simulink model "sim_Aircraft_f"  (R2016b)
settings: Solver=VariableStepAuto  StartTime=0.0  StopTime=230.0  RelTol=1e-3
values from neighbouring files (symbols this model uses):
  A = [-0.322, 0.052, 0.028, -1.12 , 0.002;       0     , 0    , 1    , -0.001,     0;       -10.6 , 0    , -2.87, 0.46  , -0.65;       6.87  , 0    , -0.04, -0.32 , -0.02;       0     , 0    , 0    , 0     ,   -10 ]    [run_task_3f.m]
  A_k = [-0.322, 0.052, 0.028, -1.12 ;       0     , 0    , 1    , -0.001;       -10.6 , 0    , -2.87, 0.46  ;       6.87  , 0    , -0.04, -0.32]    [run_task_3f.m]
  B = [0 0 0 0 10]'    [run_task_3f.m]
  B_k = [0.002, 0, -0.65, -0.2]'    [run_task_3f.m]
  C = [0 0 0 1 0;       0 0 1 0 0;       1 0 0 0 0;       0 1 0 0 0]    [run_task_3f.m]
  C_k = [0 1 0 0;       0 0 1 0;       0 0 0 1]    [run_task_3f.m]
  D = zeros(4,1)    [run_task_3f.m]
  D_k = zeros(3,1)    [run_task_3f.m]
  k_d_phi = f_kd(zp, wp)    [run_task_3f.m]
  k_i_chi = V_g/g * wx^2    [run_task_3f.m]
  k_i_phi = 0    [run_task_3f.m]
  k_p_chi = V_g/g * 2*zx*wx    [run_task_3f.m]
  k_p_phi = -5/3    (= -1.66666666667)    [run_task_3f.m]
  Ts = 1/10    (= 0.1)    [run_task_3f.m]
libraries: simulink_extras x11
settings Model: Creator=helene  LastModifiedBy=helene
settings ConfigComp: DVTestSuiteOptimization=CombinedObjectives (Nonlinear Extended)  DVDetectFloatOverflow=off

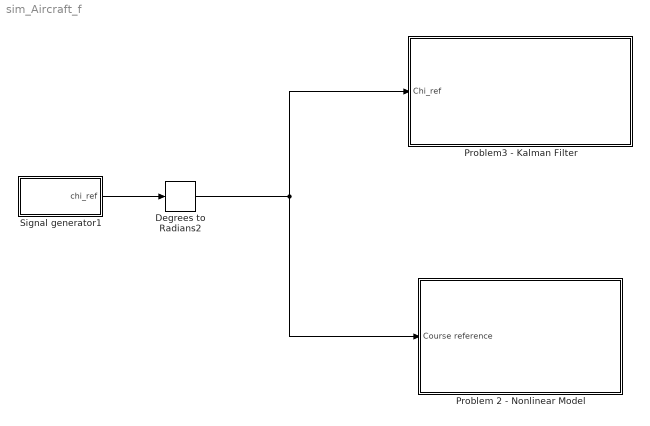
== system sim_Aircraft_f ==
  Degrees to Radians2 : simulink_extras/Transformations/Degrees to Radians
  Problem 2 - Nonlinear Model : Subsystem
  Problem3 - Kalman Filter : Subsystem
  Signal generator1 : Subsystem
  wires:
  Signal generator1/1(chi_ref) -> Degrees to Radians2/1
  Degrees to Radians2/1 -> Problem3 - Kalman Filter/1(Chi_ref), Problem 2 - Nonlinear Model/1(Course reference)

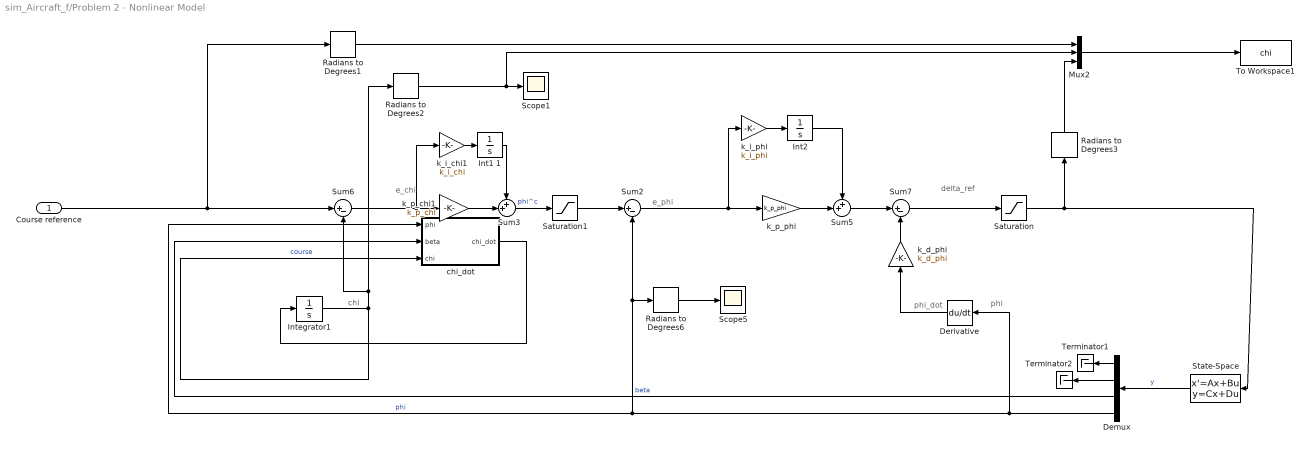
== system sim_Aircraft_f/Problem 2 - Nonlinear Model ==
  note: e_chi
  note: chi
  note: phi_dot
  note: e_phi
  note: phi
  note: delta_ref
  Course reference : Inport
  Demux : Demux
  Derivative : Derivative
  Int1 1 : Integrator  UpperSaturationLimit=0.15  LowerSaturationLimit=-0.15
  "Int2 " : Integrator
  Integrator1 : Integrator
  Mux2 : Mux  Inputs=3
  Radians to Degrees{1..3,6} (4 alike) : simulink_extras/Transformations/Radians to Degrees
  Saturation : Saturate  UpperLimit=25*deg2rad  LowerLimit=-25*deg2rad
  Saturation1 : Saturate  UpperLimit=4000*deg2rad  LowerLimit=-4000*deg2rad
  Scope1 : Scope
  Scope5 : Scope
  State-Space : StateSpace  A=A  B=B  C=C  D=D  X0=0
  Sum2 : Sum  Inputs=|+-
  Sum3 : Sum  Inputs=++|
  Sum5 : Sum  Inputs=++|
  Sum6 : Sum  Inputs=|+-
  Sum7 : Sum  Inputs=|+-
  Terminator1 : Terminator
  Terminator2 : Terminator
  To Workspace1 : ToWorkspace  VariableName=chi  SaveFormat=Timeseries  SampleTime=-1
  chi_dot : MATLAB Function  TreatAsAtomicUnit=on
  k_d_phi : Gain  Gain=k_d_phi
  k_i_chi1 : Gain  Gain=k_i_chi
  k_i_phi : Gain  Gain=k_i_phi
  k_p_chi1 : Gain  Gain=k_p_chi
  "k_p_phi " : Gain  Gain=k_p_phi
  wires:
  "Int2 "/1 -> Sum5/1
  Derivative/1 -> k_d_phi/1
  k_d_phi/1 -> Sum7/2
  Radians to Degrees2/1 -> Mux2/2, Scope1/1
  chi_dot/1(chi_dot) -> Integrator1/1
  Radians to Degrees6/1 -> Scope5/1
  Demux/4 -> Derivative/1, Radians to Degrees6/1, Sum2/2, chi_dot/1(phi)  "phi"
  k_i_phi/1 -> "Int2 "/1
  State-Space/1 -> Demux/1  "y"
  Radians to Degrees3/1 -> Mux2/3
  Sum3/1 -> Saturation1/1  "phi^c"
  "k_p_phi "/1 -> Sum5/2
  Course reference/1 -> Sum6/1, Radians to Degrees1/1
  k_i_chi1/1 -> Int1 1/1
  Demux/3 -> chi_dot/2(beta)  "beta"
  Sum2/1 -> k_i_phi/1, "k_p_phi "/1
  Int1 1/1 -> Sum3/1
  Mux2/1 -> To Workspace1/1
  Integrator1/1 -> chi_dot/3(chi), Radians to Degrees2/1, Sum6/2  "course"
  k_p_chi1/1 -> Sum3/2
  Saturation1/1 -> Sum2/1
  Sum5/1 -> Sum7/1
  Sum7/1 -> Saturation/1
  Saturation/1 -> State-Space/1, Radians to Degrees3/1
  Sum6/1 -> k_i_chi1/1, k_p_chi1/1
  Demux/1 -> Terminator1/1
  Demux/2 -> Terminator2/1
  Radians to Degrees1/1 -> Mux2/1

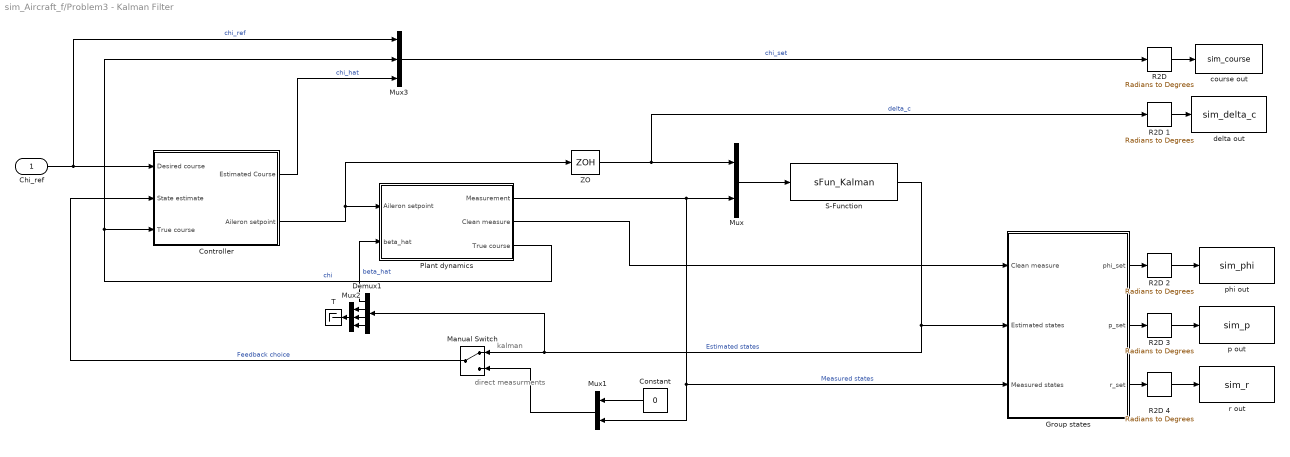
== system sim_Aircraft_f/Problem3 - Kalman Filter ==
  note: direct
      | measurments
  note: kalman
  Chi_ref : Inport
  Constant : Constant  Value=0
  Controller : Subsystem
  Demux1 : Demux
  Group states : Subsystem
  Manual Switch : ManualSwitch
  Mux : Mux  Inputs=2
  Mux1 : Mux  Inputs=2
  Mux2 : Mux  Inputs=3
  Mux3 : Mux  Inputs=3
  "Plant dynamics " : Subsystem
  R2D : simulink_extras/Transformations/Radians to Degrees
  R2D {1..4} (4 alike) : simulink_extras/Transformations/Radians to Degrees
  S-Function : S-Function  FunctionName=sFun_Kalman  Parameters=data  SFunctionDeploymentMode=off  EnableBusSupport=off
  T : Terminator
  ZO : ZeroOrderHold  SampleTime=Ts
  course out : ToWorkspace  VariableName=sim_course  SaveFormat=Timeseries  SampleTime=-1
  delta out : ToWorkspace  VariableName=sim_delta_c  SaveFormat=Timeseries  SampleTime=-1
  p out : ToWorkspace  VariableName=sim_p  SaveFormat=Timeseries  SampleTime=-1
  "phi out " : ToWorkspace  VariableName=sim_phi  SaveFormat=Timeseries  SampleTime=-1
  "r out " : ToWorkspace  VariableName=sim_r  SaveFormat=Timeseries  SampleTime=-1
  wires:
  "Plant dynamics "/3(True course) -> Mux3/2, Controller/3(True course)  "chi"
  Controller/2(Aileron setpoint) -> ZO/1, "Plant dynamics "/1("Aileron setpoint ")
  Chi_ref/1 -> Mux3/1, Controller/1(Desired course)  "chi_ref"
  Mux/1 -> S-Function/1
  ZO/1 -> R2D 1/1, Mux/1  "delta_c"
  Constant/1 -> Mux1/1
  S-Function/1 -> Manual Switch/1, Demux1/1, Group states/2(Estimated states)  "Estimated states"
  Mux1/1 -> Manual Switch/2
  Manual Switch/1 -> Controller/2(State estimate)  "Feedback choice"
  R2D 1/1 -> delta out/1
  Mux3/1 -> R2D/1  "chi_set"
  R2D/1 -> course out/1
  Controller/1(Estimated Course) -> Mux3/3  "chi_hat"
  "Plant dynamics "/1(Measurement) -> Mux1/2, Group states/3(Measured states), Mux/2  "Measured states"
  Demux1/1 -> "Plant dynamics "/2("beta_hat ")  "beta_hat"
  Demux1/2 -> Mux2/1
  Demux1/3 -> Mux2/2
  Demux1/4 -> Mux2/3
  Mux2/1 -> T/1
  "Plant dynamics "/2("Clean measure ") -> Group states/1(Clean measure)
  Group states/1(phi_set) -> R2D 2/1
  Group states/2(p_set) -> R2D 3/1
  Group states/3("r_set ") -> R2D 4/1
  R2D 2/1 -> "phi out "/1
  R2D 3/1 -> p out/1
  R2D 4/1 -> "r out "/1

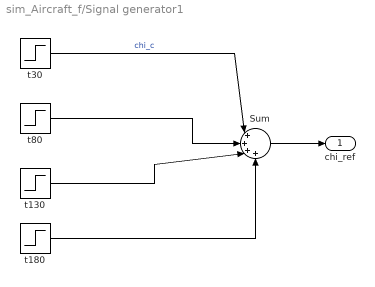
== system sim_Aircraft_f/Signal generator1 ==
  Sum : Sum  Inputs=|++++
  t130 : Step  Time=130  After=-15  SampleTime=0
  t180 : Step  Time=180  After=-10  SampleTime=0
  t30 : Step  Time=30  After=15  SampleTime=0
  "t80 " : Step  Time=80  After=10  SampleTime=0
  chi_ref : Outport
  wires:
  Sum/1 -> chi_ref/1
  t30/1 -> Sum/1  "chi_c"
  "t80 "/1 -> Sum/2
  t130/1 -> Sum/3
  t180/1 -> Sum/4

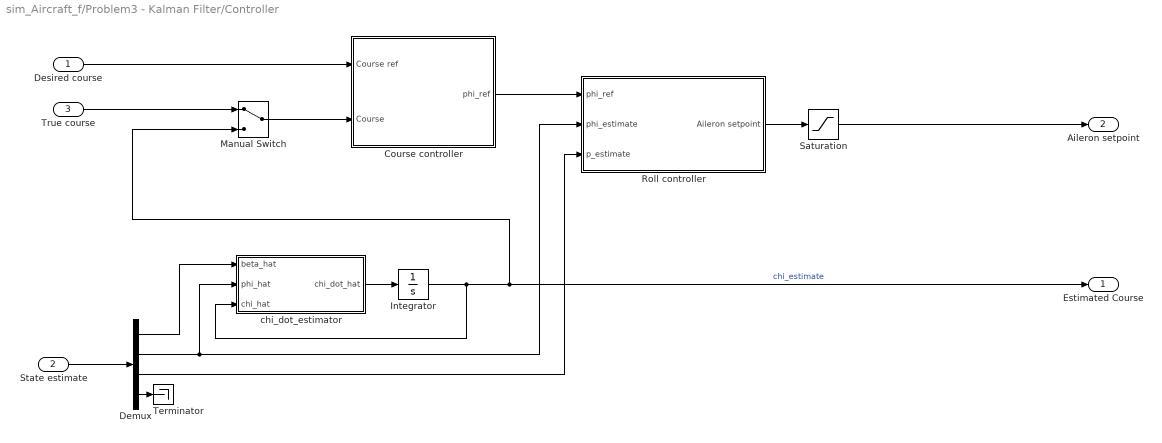
== system sim_Aircraft_f/Problem3 - Kalman Filter/Controller ==
  Desired course : Inport
  State estimate : Inport  Port=2
  True course : Inport  Port=3
  Course controller : Subsystem
  Demux : Demux
  Integrator : Integrator
  Manual Switch : ManualSwitch
  Roll controller : Subsystem
  Saturation : Saturate  UpperLimit=25*deg2rad  LowerLimit=-25*deg2rad
  Terminator : Terminator
  chi_dot_estimator : MATLAB Function  TreatAsAtomicUnit=on
  Estimated Course : Outport
  Aileron setpoint : Outport  Port=2
  wires:
  State estimate/1 -> Demux/1
  Course controller/1(phi_ref) -> Roll controller/1(phi_ref)
  Demux/3 -> Roll controller/3(p_estimate)
  Demux/2 -> Roll controller/2(phi_estimate), chi_dot_estimator/2(phi_hat)
  Desired course/1 -> Course controller/1(Course ref)
  chi_dot_estimator/1(chi_dot_hat) -> Integrator/1
  Demux/1 -> chi_dot_estimator/1(beta_hat)
  Demux/4 -> Terminator/1
  Roll controller/1(Aileron setpoint) -> Saturation/1
  Saturation/1 -> Aileron setpoint/1
  Integrator/1 -> Manual Switch/2, Estimated Course/1, chi_dot_estimator/3(chi_hat)  "chi_estimate"
  True course/1 -> Manual Switch/1
  Manual Switch/1 -> Course controller/2("Course ")

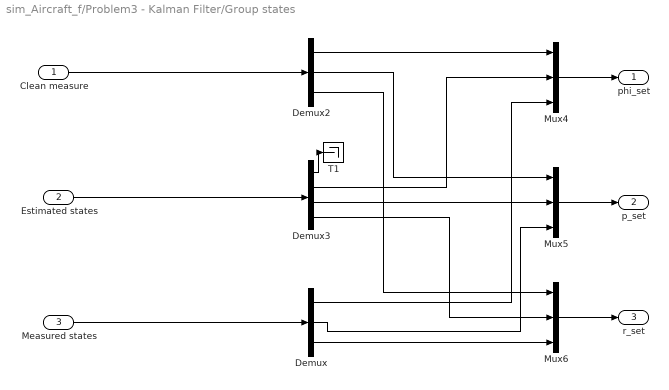
== system sim_Aircraft_f/Problem3 - Kalman Filter/Group states ==
  Clean measure : Inport
  Estimated states : Inport  Port=2
  Measured states : Inport  Port=3
  Demux : Demux  Outputs=3
  Demux2 : Demux  Outputs=3
  Demux3 : Demux
  Mux4 : Mux  Inputs=3
  Mux5 : Mux  Inputs=3
  Mux6 : Mux  Inputs=3
  T1 : Terminator
  phi_set : Outport
  p_set : Outport  Port=2
  "r_set " : Outport  Port=3
  wires:
  Demux/1 -> Mux4/3
  Estimated states/1 -> Demux3/1
  Mux5/1 -> p_set/1
  Demux3/3 -> Mux5/2
  Demux/2 -> Mux5/3
  Mux4/1 -> phi_set/1
  Demux3/4 -> Mux6/2
  Demux3/1 -> T1/1
  Demux2/1 -> Mux4/1
  Demux2/3 -> Mux6/1
  Demux/3 -> Mux6/3
  Measured states/1 -> Demux/1
  Demux2/2 -> Mux5/1
  Clean measure/1 -> Demux2/1
  Mux6/1 -> "r_set "/1
  Demux3/2 -> Mux4/2

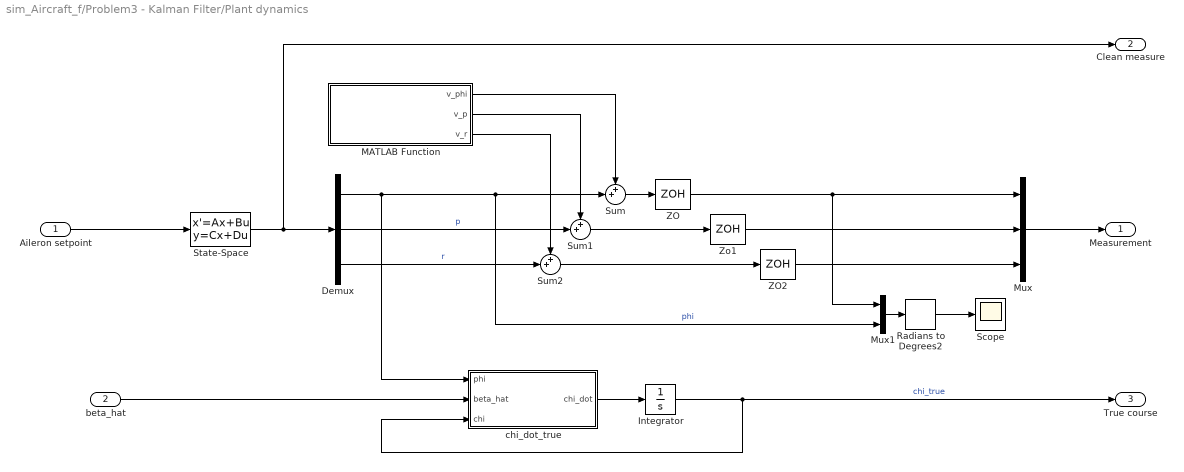
== system sim_Aircraft_f/Problem3 - Kalman Filter/Plant dynamics  ==
  "Aileron setpoint " : Inport
  "beta_hat " : Inport  Port=2
  Demux : Demux  Outputs=3
  Integrator : Integrator
  MATLAB Function : MATLAB Function  TreatAsAtomicUnit=on
  Mux : Mux  Inputs=3
  Mux1 : Mux  Inputs=2
  Radians to Degrees2 : simulink_extras/Transformations/Radians to Degrees
  Scope : Scope
  State-Space : StateSpace  A=A_k  B=B_k  C=C_k  D=D_k  X0=0
  Sum : Sum  Inputs=++|
  Sum1 : Sum  Inputs=++|
  Sum2 : Sum  Inputs=++|
  ZO : ZeroOrderHold  SampleTime=Ts
  ZO2 : ZeroOrderHold  SampleTime=Ts
  "Zo1 " : ZeroOrderHold  SampleTime=Ts
  chi_dot_true : MATLAB Function  TreatAsAtomicUnit=on
  Measurement : Outport
  "Clean measure " : Outport  Port=2
  True course : Outport  Port=3
  wires:
  "Aileron setpoint "/1 -> State-Space/1
  State-Space/1 -> Demux/1, "Clean measure "/1
  Mux/1 -> Measurement/1
  Demux/1 -> chi_dot_true/1(phi), Mux1/2, Sum/2  "phi"
  Sum/1 -> ZO/1
  Sum1/1 -> "Zo1 "/1
  Sum2/1 -> ZO2/1
  Demux/2 -> Sum1/2  "p"
  Demux/3 -> Sum2/2  "r"
  MATLAB Function/2(v_p) -> Sum1/1
  MATLAB Function/3(v_r) -> Sum2/1
  MATLAB Function/1(v_phi) -> Sum/1
  Mux1/1 -> Radians to Degrees2/1
  Radians to Degrees2/1 -> Scope/1
  ZO/1 -> Mux1/1, Mux/1
  "Zo1 "/1 -> Mux/2
  ZO2/1 -> Mux/3
  chi_dot_true/1(chi_dot) -> Integrator/1
  Integrator/1 -> True course/1, chi_dot_true/3(chi)  "chi_true"
  "beta_hat "/1 -> chi_dot_true/2(beta_hat)

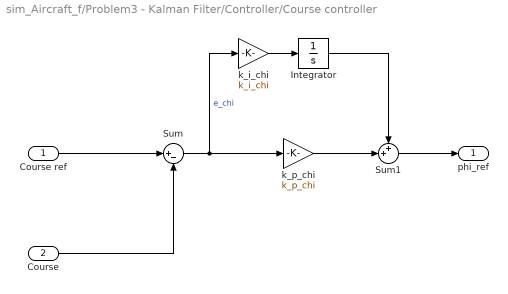
== system sim_Aircraft_f/Problem3 - Kalman Filter/Controller/Course controller ==
  Course ref : Inport
  "Course " : Inport  Port=2
  Integrator : Integrator  LimitOutput=on  UpperSaturationLimit=0.15  LowerSaturationLimit=-0.15
  Sum : Sum  Inputs=|+-
  Sum1 : Sum  Inputs=++|
  k_i_chi : Gain  Gain=k_i_chi
  k_p_chi : Gain  Gain=k_p_chi
  phi_ref : Outport
  wires:
  Course ref/1 -> Sum/1
  "Course "/1 -> Sum/2
  Sum/1 -> k_i_chi/1, k_p_chi/1  "e_chi"
  k_p_chi/1 -> Sum1/2
  Sum1/1 -> phi_ref/1
  k_i_chi/1 -> Integrator/1
  Integrator/1 -> Sum1/1

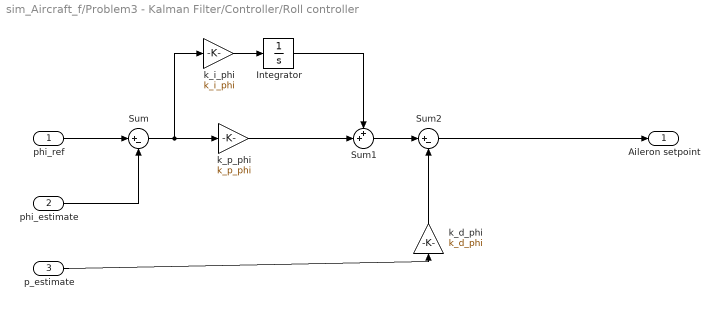
== system sim_Aircraft_f/Problem3 - Kalman Filter/Controller/Roll controller ==
  phi_ref : Inport
  phi_estimate : Inport  Port=2
  p_estimate : Inport  Port=3
  Integrator : Integrator
  Sum : Sum  Inputs=|+-
  Sum1 : Sum  Inputs=++|
  Sum2 : Sum  Inputs=|+-
  k_d_phi : Gain  Gain=k_d_phi
  k_i_phi : Gain  Gain=k_i_phi
  k_p_phi : Gain  Gain=k_p_phi
  Aileron setpoint : Outport
  wires:
  phi_ref/1 -> Sum/1
  phi_estimate/1 -> Sum/2
  k_i_phi/1 -> Integrator/1
  Sum/1 -> k_i_phi/1, k_p_phi/1
  k_p_phi/1 -> Sum1/2
  Integrator/1 -> Sum1/1
  Sum1/1 -> Sum2/1
  k_d_phi/1 -> Sum2/2
  p_estimate/1 -> k_d_phi/1
  Sum2/1 -> Aileron setpoint/1

== matlab function sim_Aircraft_f/Problem 2 - Nonlinear Model/chi_dot ==
  data: phi input; beta input; chi input; chi_dot output
function chi_dot = fcn(phi,beta, chi)

d = 2 * pi/180;
g = 9.81; % [m/s^2] gravity
V_g = 637/3.6 ; % [m/s] Speed over ground (637 [km/h]) 

psi  = chi - beta;


chi_dot = g/V_g * tan(phi+d) *cos(chi - psi);

== matlab function sim_Aircraft_f/Problem3 - Kalman Filter/Plant dynamics /MATLAB Function ==
  data: v_phi output; v_p output; v_r output
function [v_phi, v_p, v_r] = measurementNoise()
deg2rad = pi/180;

var_phi = (2*deg2rad)^2;
var_p   = (0.5*deg2rad)^2;
var_r   = (0.2*deg2rad)^2;

v_phi = sqrt(var_phi)*randn();
v_p   = sqrt(var_p)*randn();
v_r   = sqrt(var_r)*randn();

== matlab function sim_Aircraft_f/Problem3 - Kalman Filter/Controller/chi_dot_estimator ==
  data: beta_hat input; phi_hat input; chi_hat input; chi_dot_hat output
function chi_dot_hat = fcn(beta_hat,phi_hat, chi_hat)

d = 0*2 * pi/180; % Cannot know anything about the bias in the estimator?
g = 9.81; % [m/s^2] gravity
V_g = 637/3.6 ; % [m/s] Speed over ground (637 [km/h]) 

psi_hat  = chi_hat - beta_hat;


chi_dot_hat = g/V_g * tan(phi_hat+d) *cos(chi_hat - psi_hat);

== matlab function sim_Aircraft_f/Problem3 - Kalman Filter/Plant dynamics /chi_dot_true ==
  data: phi input; beta_hat input; chi input; chi_dot output
function chi_dot = fcn(phi, beta_hat, chi)

d = 2 * pi/180;
g = 9.81; % [m/s^2] gravity
V_g = 637/3.6 ; % [m/s] Speed over ground (637 [km/h]) 

psi_hat  = chi - beta_hat;


chi_dot = g/V_g * tan(phi+d) *cos(chi - psi_hat);
